simulink model "EVCS_APF_V2G"  (R2024b)
settings: Solver=ode23tb  StartTime=0.0  StopTime=Tstop  MaxStep=1e-5  RelTol=1e-4
PreLoadFcn:
  | model_params
values from neighbouring files (symbols this model uses):
  alpha_lpf = Ts/(tau_lpf+Ts)    (= 0.000125647916761)    [model_params.m]
  Cdc = 3000e-6    (= 0.003)    [model_params.m]
  Cpv = 500e-6    (= 0.0005)    [model_params.m]
  Crf = 20e-6    (= 2e-05)    [model_params.m]
  duty_fix = 0.58    [model_params.m]
  ev_enable = 1    [model_params.m]
  ev_openloop = 0    [model_params.m]
  fgrid = 50    [model_params.m]
  fsw = 10e3    (= 10000)    [model_params.m]
  HB = 0.35    [model_params.m]
  HystSign = -1    [model_params.m]
  Iev_ref = 20    [model_params.m]
  iev_sign = 1    [model_params.m]
  Irr0 = 1000    [model_params.m]
  Irr1 = 700    [model_params.m]
  Ki_dc = 24.6    [model_params.m]
  Ki_ev = 20    [model_params.m]
  Kp_dc = 1.85    [model_params.m]
  Kp_ev = 0.01    [model_params.m]
  Kpu = 1/(VLL*sqrt(2/3))    [model_params.m]
  Lboost = 1.5e-3    (= 0.0015)    [model_params.m]
  Ldc_nl = 20e-3    (= 0.02)    [model_params.m]
  Lev = 5e-3    (= 0.005)    [model_params.m]
  Lf = 1.5e-3    (= 0.0015)    [model_params.m]
  Ls_src = 0.15e-3    (= 0.00015)    [model_params.m]
  Rdc_nl = 10    [model_params.m]
  Rev = 0.2    [model_params.m]
  Rrf = 5    [model_params.m]
  Rs_src = 0.1    [model_params.m]
  t_irr = 0.20    (= 0.2)    [model_params.m]
  t_v2g = 0.30    (= 0.3)    [model_params.m]
  Tcell = 25    [model_params.m]
  Ts = evalin('base','Ts')    [apf_metrics.m]    (also in complexity_analysis.m; harmonic_diagnose.m; model_params.m = 2e-06)
  Vdc_ref = 750    [model_params.m]    (also in pso_tune.m = evalin('base','Vdc_ref'); pso_tune_short.m = evalin('base','Vdc_ref'))
  VLL = 415    [model_params.m]
undefined symbols (not defined in the file or in its folder): Ion, Lithium
libraries: spsSeriesRLCBranchLib x5, spsIGBTDiodeLib x3, spsUniversalBridgeLib x2, spsCurrentMeasurementLib x2, spsThreePhaseSeriesRLCBranchLib x2, spsThreePhaseVIMeasurementLib x2, slpidlib x2, spsVoltageMeasurementLib x2, spsDiodeLib x1, spsBatteryLib x1, spsThreePhaseSourceLib x1, spsThreePhaseSeriesRLCLoadLib x1
settings Model: Creator=dines  LastModifiedBy=dines

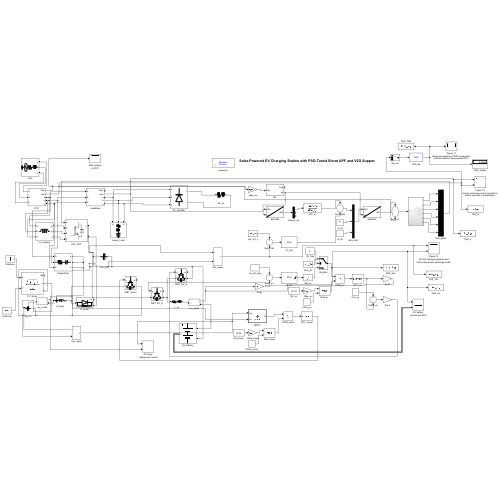
[thumbnail: Simulink's stored preview of the top-level diagram]
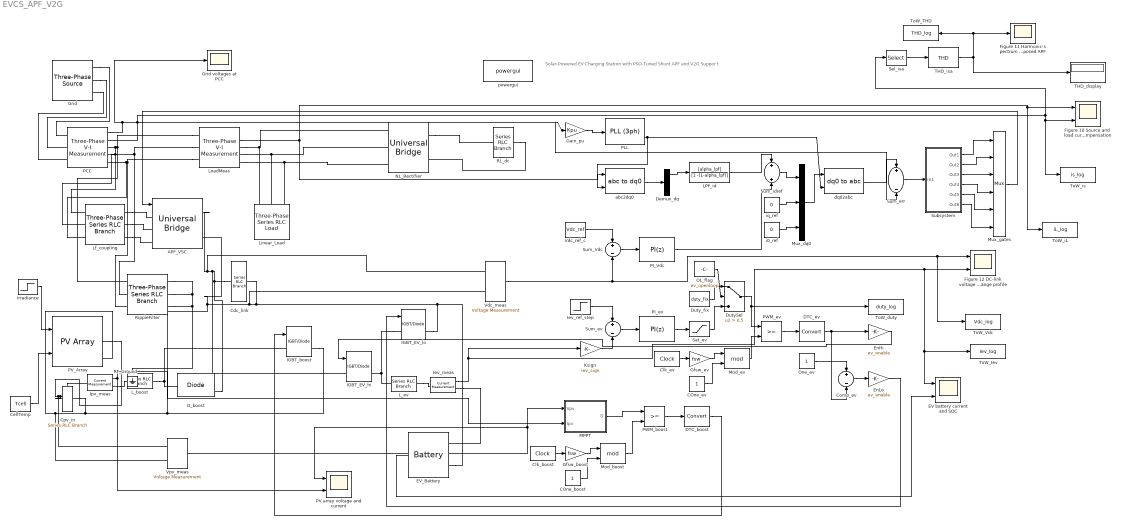
== system EVCS_APF_V2G ==
  note: Solar-Powered EV Charging Station with PSO-Tuned Shunt APF and V2G Suppor t
  APF_VSC : spsUniversalBridgeLib/Universal Bridge  Arms=3  SnubberResistance=1e5  SnubberCapacitance=inf  Device=IGBT / Diodes  Ron=1e-3  Lon=0  ForwardVoltages="[  0  0  ]"  ForwardVoltage=0  GTOparameters=[ 10e-6 , 20e-6 ]  IGBTparameters=[ 1e-6 , 2e-6 ]  Measurements=None  Measurements_2=None  converterType=Rectifier
  COne_boost : Constant
  COne_ev : Constant
  Cdc_link : spsSeriesRLCBranchLib/Series RLC Branch  LConnTagsString=__new0  RConnTagsString=__new0  BranchType=C  Resistance=1  Inductance=1e-3  SetiL0=off  InitialCurrent=0  Capacitance=Cdc  Setx0=off  InitialVoltage=0  Measurements=None
  CellTemp : Constant  Value=Tcell
  Clk_boost : DigitalClock  SampleTime=Ts
  Clk_ev : DigitalClock  SampleTime=Ts
  Comp_ev : Sum  Inputs=+-
  Cpv_in : spsSeriesRLCBranchLib/Series RLC Branch  LConnTagsString=__new0  RConnTagsString=__new0  BranchType=C  Resistance=1  Inductance=1e-3  SetiL0=off  InitialCurrent=0  Capacitance=Cpv  Setx0=off  InitialVoltage=0  Measurements=None
  DTC_boost : DataTypeConversion  SaturateOnIntegerOverflow=off  RndMeth=Floor
  DTC_ev : DataTypeConversion  SaturateOnIntegerOverflow=off  RndMeth=Floor
  D_boost : spsDiodeLib/Diode  Ron=0.001  Lon=0  Vf=0.8  IC=0  UseSnubber=0  Rs=500  Cs=250e-9  Measurements=on
  Demux_dq : Demux  Outputs=3
  DutySel : Switch  Criteria=u2 > Threshold  Threshold=0.5  SaturateOnIntegerOverflow=off  InputSameDT=off
  Duty_fix : Constant  Value=duty_fix
  EV battery current and SOC : Scope  NumInputPorts=2
  EV_Battery : spsBatteryLib/Battery  BatType=Lithium-Ion  NomV=Vbatt  NomQ=Qbatt  SOC=SOC0  Batt_Tr=30  PresetModel=on  MaxQ=40  MinV=270  FullV=419.0354  Dis_rate=17.3913  R=0.09  Normal_OP=36.1739  expZone="[388.9389      1.965217]"
  EnHi : Gain  Gain=ev_enable
  EnLo : Gain  Gain=ev_enable
  Figure 10 Source and load current waveforms before and after compensation : Scope  NumInputPorts=2
  Figure 11 Harmonic-spectrum (THD) comparison with and without the proposed APF : Scope
  Figure 12 DC-link voltage regulation and V2G active-power exchange profile : Scope  NumInputPorts=2
  Gain_pu : Gain  Gain=Kpu
  Gfsw_boost : Gain  Gain=fsw
  Gfsw_ev : Gain  Gain=fsw
  Grid : spsThreePhaseSourceLib/Three-Phase Source  InternalConnection=Yg  VoltagePhases=off  Voltage=VLL  PhaseAngle=0  Voltage_phases=[25e3 25e3 25e3]/sqrt(3)  PhaseAngles_phases=[0 -120 +120]  Frequency=fgrid  NonIdealSource=on  SpecifyImpedance=off  Resistance=Rs_src  Inductance=Ls_src  ShortCircuitLevel=100e6  BaseVoltage=25e3  XRratio=7  BusType=swing  Pref=10e3  Qref=0  Prefabc=[10e3, 10e3, 10e3]  Qrefabc=[0, 0, 0]  Qmin=-inf  Qmax=inf
  Grid voltages at PCC : Scope
  IGBT_EV_hi : spsIGBTDiodeLib/IGBT//Diode  Ron=1e-3  Rs=1e5  Cs=inf  Measurements=on
  IGBT_EV_lo : spsIGBTDiodeLib/IGBT//Diode  Ron=1e-3  Rs=1e5  Cs=inf  Measurements=on
  IGBT_boost : spsIGBTDiodeLib/IGBT//Diode  Ron=1e-3  Rs=1e5  Cs=inf  Measurements=on
  Iev_meas : spsCurrentMeasurementLib/Current Measurement  PhasorSimulation=off  OutputType=Complex  PSBequivalent=0
  Iev_ref_step : Step  Time=t_v2g  Before=Iev_ref  After=-Iev_ref  SampleTime=0
  Ipv_meas : spsCurrentMeasurementLib/Current Measurement  PhasorSimulation=off  OutputType=Complex  PSBequivalent=0
  Irradiance : Step  Time=t_irr  Before=Irr0  After=Irr1  SampleTime=0
  Ksign : Gain  Gain=iev_sign
  LPF_id : DiscreteTransferFcn  Numerator=[alpha_lpf]  Denominator=[1 -(1-alpha_lpf)]  SampleTime=Ts
  L_boost : spsSeriesRLCBranchLib/Series RLC Branch  LConnTagsString=__new0  RConnTagsString=__new0  BranchType=L  Resistance=1  Inductance=Lboost  SetiL0=off  InitialCurrent=0  Capacitance=1e-6  Setx0=off  InitialVoltage=0  Measurements=None
  L_ev : spsSeriesRLCBranchLib/Series RLC Branch  LConnTagsString=__new0  RConnTagsString=__new0  BranchType=RL  Resistance=Rev  Inductance=Lev  SetiL0=off  InitialCurrent=0  Capacitance=1e-6  Setx0=off  InitialVoltage=0  Measurements=None
  Lf_coupling : spsThreePhaseSeriesRLCBranchLib/Three-Phase Series RLC Branch  LConnTagsString=A|B|C  RConnTagsString=A|B|C  BranchType=L  Resistance=1  Inductance=Lf  Capacitance=1e-6  Measurements=None
  Linear_Load : spsThreePhaseSeriesRLCLoadLib/Three-Phase Series RLC Load  LConnTagsString=A|B|C  Configuration=Y (grounded)  NominalVoltage=VLL  Vabc=[1e3 1e3 1e3]  Vabcp=[1e3 1e3 1e3]  NominalFrequency=fgrid  UnbalancedPower=off  ActivePower=Plin  InductivePower=100  CapacitivePower=100  Pabc=[10e3 9e3 11e3]  QLabc=[100 90 110]  QCabc=[100 90 110]  Pabcp=[10e3 9e3 11e3]  QLabcp=[100 90 110]  QCabcp=[100 90 110]  Measurements=None  LoadType=constant Z
  LoadMeas : spsThreePhaseVIMeasurementLib/Three-Phase V-I Measurement  VoltageMeasurement=phase-to-ground  SetLabelV=off  LabelV=Vabc  Vpu=off  VpuLL=off  CurrentMeasurement=yes  SetLabelI=off  LabelI=Iabc  Ipu=off  Pbase=100e6  Vbase=500e3  OutputType=Complex  PhasorSimulation=off  PSBequivalent=0
  MPPT : MATLAB Function  TreatAsAtomicUnit=on
  Mod_boost : Math  Operator=mod
  Mod_ev : Math  Operator=mod
  Mux_dq0 : Mux  Inputs=3
  Mux_gates : Mux  Inputs=6
  NL_Rectifier : spsUniversalBridgeLib/Universal Bridge  Arms=3  SnubberResistance=1e5  SnubberCapacitance=inf  Device=Diodes  Ron=1e-3  Lon=0  ForwardVoltages="[  0  0  ]"  ForwardVoltage=0  GTOparameters=[ 10e-6 , 20e-6 ]  IGBTparameters=[ 1e-6 , 2e-6 ]  Measurements=None  Measurements_2=None  converterType=Rectifier
  OL_flag : Constant  Value=ev_openloop
  One_ev : Constant
  PCC : spsThreePhaseVIMeasurementLib/Three-Phase V-I Measurement  VoltageMeasurement=phase-to-ground  SetLabelV=off  LabelV=Vabc  Vpu=off  VpuLL=off  CurrentMeasurement=yes  SetLabelI=off  LabelI=Iabc  Ipu=off  Pbase=100e6  Vbase=500e3  OutputType=Complex  PhasorSimulation=off  PSBequivalent=0
  PI_Vdc : slpidlib/PID Controller  Controller=PI  Form=Parallel  TimeDomain=Discrete-time  UseExternalTs=off  SampleTime=Ts  IntegratorMethod=Forward Euler  FilterMethod=Forward Euler  ControllerParametersSource=internal  P=Kp_dc  I=Ki_dc  UseKiTs=off  D=0  UseExternalDerivativeSource=off  N=100  UseFilter=on  TunerSelectOption=Transfer Function Based (PID Tuner App)  InitialConditionSource=internal  InitialConditionForIntegrator=0  InitialConditionForFilter=0  DifferentiatorICPrevScaledInput=0  ExternalReset=none  TrackingMode=off  Kt=1  LimitOutput=off  SatLimitsSource=internal  UpperSaturationLimit=inf  LowerSaturationLimit=-inf  LinearizeAsGain=on  AntiWindupMode=none  Kb=1  LimitIntegrator=off  UpperIntegratorSaturationLimit=inf  LowerIntegratorSaturationLimit=-inf  POutMin=[]  POutMax=[]  IOutMin=[]  IOutMax=[]  DOutMin=[]  DOutMax=[]  NOutMin=[]  NOutMax=[]  SumOutMin=[]  SumOutMax=[]  SaturationOutMin=[]  SaturationOutMax=[]  PParamMin=[]  PParamMax=[]  IParamMin=[]  IParamMax=[]  DParamMin=[]  DParamMax=[]  NParamMin=[]  NParamMax=[]  KbParamMin=[]  KbParamMax=[]  KtParamMin=[]  KtParamMax=[]  KbOutMin=[]  KbOutMax=[]  KtOutMin=[]  KtOutMax=[]  IntegratorOutMin=[]  IntegratorOutMax=[]  FilterOutMin=[]  FilterOutMax=[]  SumI1OutMin=[]  SumI1OutMax=[]  SumI2OutMin=[]  SumI2OutMax=[]  SumI3OutMin=[]  SumI3OutMax=[]  SumI4OutMin=[]  SumI4OutMax=[]  SumDOutMin=[]  SumDOutMax=[]  DifferentiatorOutMin=[]  DifferentiatorOutMax=[]  FilterDiffOutCoefMin=[]  FilterDiffOutCoefMax=[]  ReciprocalOutMin=[]  ReciprocalOutMax=[]  SumDenOutMin=[]  SumDenOutMax=[]  SumNumOutMin=[]  SumNumOutMax=[]  DivideOutMin=[]  DivideOutMax=[]  UdiffTsProdOutMin=[]  UdiffTsProdOutMax=[]  NTsProdOutMin=[]  NTsProdOutMax=[]  UintegralTsProdOutMin=[]  UintegralTsProdOutMax=[]  UngainTsProdOutMin=[]  UngainTsProdOutMax=[]  ClampingZeroOutDataTypeStr=Inherit: Inherit via back propagation  ClampingZeroOutMin=[]  ClampingZeroOutMax=[]  FilterDenConstantOutDataTypeStr=Inherit: Inherit via back propagation  FilterDenConstantOutMin=[]  FilterDenConstantOutMax=[]  PCopyOutDataTypeStr=Inherit: Inherit via back propagation  PCopyOutMin=[]  PCopyOutMax=[]  NCopyOutDataTypeStr=Inherit: Inherit via back propagation  NCopyOutMin=[]  NCopyOutMax=[]  IntegratorContinuousStateAttributes=''  IntegratorStateMustResolveToSignalObject=off  IntegratorRTWStateStorageClass=Auto  FilterContinuousStateAttributes=''  FilterStateMustResolveToSignalObject=off  FilterRTWStateStorageClass=Auto  ParallelPVariant=InternalParameters  IdealPVariant=Disabled  IVariant=InternalParameters  DVariant=Disabled  IntegratorVariant=Discrete  SatVariant=Disabled  AWVariant=Passthrough  PCopyVariant=Disabled  TRVariant=Disabled  FdbkBlocksVariant=Forward  IdealPFdbkVariant=Disabled  SatFdbkVariant=Disabled  DerivativeFilterVariant=Disabled  NVariant=Disabled  NCopyVariant=Disabled_SignalSpec  FilterICVariant=Disabled  IntegratorICVariant=InternalICs  ExternalResetVariant=Disabled  TRSumVariant=Passthrough  SumFdbkVariant=Disabled  SumVariant=Sum_PI  TsampFilterVariant=InternalTs  TsampNgainVariant=Passthrough  TsampIntegralVariant=Disabled_SignalSpec  ExternalSaturationOutDataTypeStr=Inherit: Same as second input  DerivativeSourceVariant=Disabled  PreIntVariant=InternalPreInt
  PI_ev : slpidlib/PID Controller  Controller=PI  Form=Parallel  TimeDomain=Discrete-time  UseExternalTs=off  SampleTime=Ts  IntegratorMethod=Forward Euler  FilterMethod=Forward Euler  ControllerParametersSource=internal  P=Kp_ev  I=Ki_ev  UseKiTs=off  D=0  UseExternalDerivativeSource=off  N=100  UseFilter=on  TunerSelectOption=Transfer Function Based (PID Tuner App)  InitialConditionSource=internal  InitialConditionForIntegrator=duty0  InitialConditionForFilter=0  DifferentiatorICPrevScaledInput=0  ExternalReset=none  TrackingMode=off  Kt=1  LimitOutput=on  SatLimitsSource=internal  UpperSaturationLimit=0.95  LowerSaturationLimit=0.05  LinearizeAsGain=on  AntiWindupMode=clamping  Kb=1  LimitIntegrator=off  UpperIntegratorSaturationLimit=inf  LowerIntegratorSaturationLimit=-inf  POutMin=[]  POutMax=[]  IOutMin=[]  IOutMax=[]  DOutMin=[]  DOutMax=[]  NOutMin=[]  NOutMax=[]  SumOutMin=[]  SumOutMax=[]  SaturationOutMin=[]  SaturationOutMax=[]  PParamMin=[]  PParamMax=[]  IParamMin=[]  IParamMax=[]  DParamMin=[]  DParamMax=[]  NParamMin=[]  NParamMax=[]  KbParamMin=[]  KbParamMax=[]  KtParamMin=[]  KtParamMax=[]  KbOutMin=[]  KbOutMax=[]  KtOutMin=[]  KtOutMax=[]  IntegratorOutMin=[]  IntegratorOutMax=[]  FilterOutMin=[]  FilterOutMax=[]  SumI1OutMin=[]  SumI1OutMax=[]  SumI2OutMin=[]  SumI2OutMax=[]  SumI3OutMin=[]  SumI3OutMax=[]  SumI4OutMin=[]  SumI4OutMax=[]  SumDOutMin=[]  SumDOutMax=[]  DifferentiatorOutMin=[]  DifferentiatorOutMax=[]  FilterDiffOutCoefMin=[]  FilterDiffOutCoefMax=[]  ReciprocalOutMin=[]  ReciprocalOutMax=[]  SumDenOutMin=[]  SumDenOutMax=[]  SumNumOutMin=[]  SumNumOutMax=[]  DivideOutMin=[]  DivideOutMax=[]  UdiffTsProdOutMin=[]  UdiffTsProdOutMax=[]  NTsProdOutMin=[]  NTsProdOutMax=[]  UintegralTsProdOutMin=[]  UintegralTsProdOutMax=[]  UngainTsProdOutMin=[]  UngainTsProdOutMax=[]  ClampingZeroOutDataTypeStr=Inherit: Inherit via back propagation  ClampingZeroOutMin=[]  ClampingZeroOutMax=[]  FilterDenConstantOutDataTypeStr=Inherit: Inherit via back propagation  FilterDenConstantOutMin=[]  FilterDenConstantOutMax=[]  PCopyOutDataTypeStr=Inherit: Inherit via back propagation  PCopyOutMin=[]  PCopyOutMax=[]  NCopyOutDataTypeStr=Inherit: Inherit via back propagation  NCopyOutMin=[]  NCopyOutMax=[]  IntegratorContinuousStateAttributes=''  IntegratorStateMustResolveToSignalObject=off  IntegratorRTWStateStorageClass=Auto  FilterContinuousStateAttributes=''  FilterStateMustResolveToSignalObject=off  FilterRTWStateStorageClass=Auto  ParallelPVariant=InternalParameters  IdealPVariant=Disabled  IVariant=InternalParameters  DVariant=Disabled  IntegratorVariant=Discrete  SatVariant=Enabled  AWVariant=DiscClampingParallel  PCopyVariant=Disabled  TRVariant=Disabled  FdbkBlocksVariant=Forward  IdealPFdbkVariant=Disabled  SatFdbkVariant=Disabled  DerivativeFilterVariant=Disabled  NVariant=Disabled  NCopyVariant=Disabled_SignalSpec  FilterICVariant=Disabled  IntegratorICVariant=InternalICs  ExternalResetVariant=Disabled  TRSumVariant=Passthrough  SumFdbkVariant=Disabled  SumVariant=Sum_PI  TsampFilterVariant=InternalTs  TsampNgainVariant=Passthrough  TsampIntegralVariant=Disabled_SignalSpec  ExternalSaturationOutDataTypeStr=Inherit: Same as second input  DerivativeSourceVariant=Disabled  PreIntVariant=InternalPreInt
  PLL : spsPLL3phLib/PLL (3ph)  Fmin=45  Par_Init=[0, 60]  ParK=[180, 3200, 1]  TcD=1e-4  MaxRateChangeFreq=12  FilterCutOffFreq=25  Ts=Ts  AGC=on
  PV array voltage and current : Scope  NumInputPorts=2
  PV_Array : spsPVArrayLib/PV Array  Npar=Npar  Nser=Nser  PlotType=array @ 1000 W/m2 & specified temperatures  S_vec="[ 1000  500  100 ]"  Temp_C_vec="[ 45 25  ]"  ModuleName=SunPower SPR-305E-WHT-D  PlotWhenSelected=off  Pm=305.226  Ncell=96  Voc=64.2  Isc=5.96  Vm=54.7  Im=5.58  beta_Voc_pc=-0.2727  alpha_Isc_pc=0.061745  beta_Voc=-0.17507  alpha_Isc=0.00368  IL=5.9657  I0=6.3076e-12  nI=0.94489  Rsh=393.2054  Rs=0.37428  RobustModel=off  RobustCellTemperature=313.3991  BAL=on  Tc=1e-6  Tfilter=5e-5
  PWM_boost : RelationalOperator  OutDataTypeStr=boolean  RndMeth=Simplest  InputSameDT=off
  PWM_ev : RelationalOperator  OutDataTypeStr=boolean  RndMeth=Simplest  InputSameDT=off
  RF_Ground : spsGroundLib/Ground  LConnTagsString=a
  RL_dc : spsSeriesRLCBranchLib/Series RLC Branch  LConnTagsString=__new0  RConnTagsString=__new0  BranchType=RL  Resistance=Rdc_nl  Inductance=Ldc_nl  SetiL0=off  InitialCurrent=0  Capacitance=1e-6  Setx0=off  InitialVoltage=0  Measurements=None
  RippleFilter : spsThreePhaseSeriesRLCBranchLib/Three-Phase Series RLC Branch  LConnTagsString=A|B|C  RConnTagsString=A|B|C  BranchType=RC  Resistance=Rrf  Inductance=1e-3  Capacitance=Crf  Measurements=None
  Sat_ev : Saturate  UpperLimit=0.95  LowerLimit=0.05
  Sel_isa : Selector  InputPortWidth=3  IndexOptions=Index vector (dialog)  Indices=1  OutputSizes=1
  Subsystem : Subsystem
  Sum_Vdc : Sum  Inputs=+-
  Sum_err : Sum  Inputs=+-
  Sum_ev : Sum  Inputs=+-
  Sum_idref : Sum
  THD_display : Display
  THD_isa : spsTHDLib/THD  Freq=fgrid  Ts=0
  ToW_Iev : ToWorkspace  VariableName=Iev_log  SaveFormat=Timeseries  SampleTime=-1
  ToW_THD : ToWorkspace  VariableName=THD_log  SaveFormat=Timeseries  SampleTime=-1
  ToW_Vdc : ToWorkspace  VariableName=Vdc_log  SaveFormat=Timeseries  SampleTime=-1
  ToW_duty : ToWorkspace  VariableName=duty_log  SaveFormat=Timeseries  SampleTime=-1
  ToW_iL : ToWorkspace  VariableName=iL_log  SaveFormat=Timeseries  SampleTime=-1
  ToW_is : ToWorkspace  VariableName=is_log  SaveFormat=Timeseries  SampleTime=-1
  Vdc_meas : spsVoltageMeasurementLib/Voltage Measurement  PhasorSimulation=off  OutputType=Complex  PSBequivalent=0
  Vdc_ref_c : Constant  Value=Vdc_ref
  Vpv_meas : spsVoltageMeasurementLib/Voltage Measurement  PhasorSimulation=off  OutputType=Complex  PSBequivalent=0
  abc2dq0 : spsabctodq0Lib/abc to dq0  Alignment=90 degrees behind phase A axis
  dq02abc : spsdq0toabcLib/dq0 to abc  Alignment=90 degrees behind phase A axis
  i0_ref : Constant  Value=0
  iq_ref : Constant  Value=0
  powergui : sps_lib/powergui  Priority=1  SimulationMode=Discrete  SampleTime=Ts  frequency=60  Iterations=50  frequencyindice=0  Pbase=100e6  ErrMax=1e-4  UnitsV=kV  UnitsW=MW  buscounter=0  FunctionMessages=off  echomessages=off  EnableUseOfTLC=off  CurrentSourceSwitches=off  DisableSnubberDevices=off  DisableRonSwitches=off  DisableVfSwitches=off  DisplayEquations=off  AutomaticDiscreteSolvers=off  SolverType=Tustin/Backward Euler (TBE)  Interpol=off  ExternalGateDelay=off  methode=off  Ts=100  x0status=blocks  SPID=on  SwTol=0  HookPort=off  NonlinearTolerance=1e-4  nMaxIteration=100  ContinueOnMaxIteration=off  RestoreLinks=warning  ResistiveCurrentMeasurement=off  Frange=[0:2:500]  Ylog=off  Xlog=on  ShowGrid=off  save=off  variable=ZData  structure=0  ZoomFFT=off  StartTime=0.0  cycles=1  DisplayStyle=1  fundamental=60  FreqAxis=off  MaxFrequency=1000  frequencyindicesteady=1  RmsSteady=1  display=off
  wires:
  Irradiance/1 -> PV_Array/1
  CellTemp/1 -> PV_Array/2
  PCC/1 -> Gain_pu/1, Grid voltages at PCC/1
  Gain_pu/1 -> PLL/1
  PLL/2 -> abc2dq0/2, dq02abc/2
  LoadMeas/2 -> Figure 10 Source and load current waveforms before and after compensation/1, ToW_iL/1, abc2dq0/1
  abc2dq0/1 -> Demux_dq/1
  Demux_dq/1 -> LPF_id/1
  Vdc_ref_c/1 -> Sum_Vdc/1
  Vdc_meas/1 -> Figure 12 DC-link voltage regulation and V2G active-power exchange profile/1, ToW_Vdc/1, Sum_Vdc/2
  Sum_Vdc/1 -> PI_Vdc/1
  LPF_id/1 -> Sum_idref/1
  PI_Vdc/1 -> Sum_idref/2
  Sum_idref/1 -> Mux_dq0/1
  iq_ref/1 -> Mux_dq0/2
  i0_ref/1 -> Mux_dq0/3
  Mux_dq0/1 -> dq02abc/1
  dq02abc/1 -> Sum_err/1
  PCC/2 -> Sel_isa/1, ToW_is/1, Figure 10 Source and load current waveforms before and after compensation/2, Sum_err/2
  Mux_gates/1 -> APF_VSC/1
  Vpv_meas/1 -> MPPT/1(Vpv), PV array voltage and current/1
  Ipv_meas/1 -> MPPT/2(Ipv), PV array voltage and current/2
  MPPT/1(D) -> PWM_boost/1
  Clk_boost/1 -> Gfsw_boost/1
  Gfsw_boost/1 -> Mod_boost/1
  COne_boost/1 -> Mod_boost/2
  Mod_boost/1 -> PWM_boost/2
  PWM_boost/1 -> DTC_boost/1
  DTC_boost/1 -> IGBT_boost/1
  Iev_ref_step/1 -> Sum_ev/1
  Iev_meas/1 -> ToW_Iev/1, EV battery current and SOC/1, Figure 12 DC-link voltage regulation and V2G active-power exchange profile/2, Ksign/1
  Ksign/1 -> Sum_ev/2
  Sum_ev/1 -> PI_ev/1
  PI_ev/1 -> Sat_ev/1
  Duty_fix/1 -> DutySel/1
  OL_flag/1 -> DutySel/2
  Sat_ev/1 -> DutySel/3
  DutySel/1 -> PWM_ev/1, ToW_duty/1
  Clk_ev/1 -> Gfsw_ev/1
  Gfsw_ev/1 -> Mod_ev/1
  COne_ev/1 -> Mod_ev/2
  Mod_ev/1 -> PWM_ev/2
  PWM_ev/1 -> DTC_ev/1
  One_ev/1 -> Comp_ev/1
  DTC_ev/1 -> EnHi/1, Comp_ev/2
  Comp_ev/1 -> EnLo/1
  EnHi/1 -> IGBT_EV_hi/1
  EnLo/1 -> IGBT_EV_lo/1
  Sel_isa/1 -> THD_isa/1
  THD_isa/1 -> ToW_THD/1, Figure 11 Harmonic-spectrum (THD) comparison with and without the proposed APF/1, THD_display/1
  EV_Battery/1 -> EV battery current and SOC/2
  Sum_err/1 -> Subsystem/1(In1)
  Subsystem/1(Out1) -> Mux_gates/1
  Subsystem/2(Out2) -> Mux_gates/2
  Subsystem/3(Out3) -> Mux_gates/3
  Subsystem/4(Out4) -> Mux_gates/4
  Subsystem/5(Out5) -> Mux_gates/5
  Subsystem/6(Out6) -> Mux_gates/6
  connections:
  Grid/RConn1 -- PCC/LConn1
  Grid/RConn2 -- PCC/LConn2
  Grid/RConn3 -- PCC/LConn3
  LoadMeas/LConn1 -- PCC/RConn1 -- Lf_coupling/LConn1 -- RippleFilter/LConn1
  LoadMeas/LConn2 -- PCC/RConn2 -- Lf_coupling/LConn2 -- RippleFilter/LConn2
  LoadMeas/LConn3 -- PCC/RConn3 -- Lf_coupling/LConn3 -- RippleFilter/LConn3
  LoadMeas/RConn1 -- NL_Rectifier/LConn1 -- Linear_Load/LConn1
  LoadMeas/RConn2 -- NL_Rectifier/LConn2 -- Linear_Load/LConn2
  LoadMeas/RConn3 -- NL_Rectifier/LConn3 -- Linear_Load/LConn3
  NL_Rectifier/RConn1 -- RL_dc/LConn1
  RL_dc/RConn1 -- NL_Rectifier/RConn2
  Lf_coupling/RConn1 -- APF_VSC/LConn1
  Lf_coupling/RConn2 -- APF_VSC/LConn2
  Lf_coupling/RConn3 -- APF_VSC/LConn3
  Cdc_link/LConn1 -- APF_VSC/RConn1 -- Vdc_meas/LConn1 -- IGBT_EV_hi/LConn1 -- D_boost/RConn1
  Cdc_link/RConn1 -- EV_Battery/LConn2 -- IGBT_EV_lo/RConn1 -- APF_VSC/RConn2 -- PV_Array/RConn2 -- Vpv_meas/LConn2 -- Cpv_in/RConn1 -- IGBT_boost/RConn1 -- Vdc_meas/LConn2
  Cpv_in/LConn1 -- PV_Array/RConn1 -- Vpv_meas/LConn1 -- Ipv_meas/LConn1
  Ipv_meas/RConn1 -- L_boost/LConn1
  D_boost/LConn1 -- IGBT_boost/LConn1 -- L_boost/RConn1
  IGBT_EV_lo/LConn1 -- L_ev/LConn1 -- IGBT_EV_hi/RConn1
  L_ev/RConn1 -- Iev_meas/LConn1
  Iev_meas/RConn1 -- EV_Battery/LConn1
  RippleFilter/RConn1 -- RF_Ground/LConn1 -- RippleFilter/RConn3 -- RippleFilter/RConn2

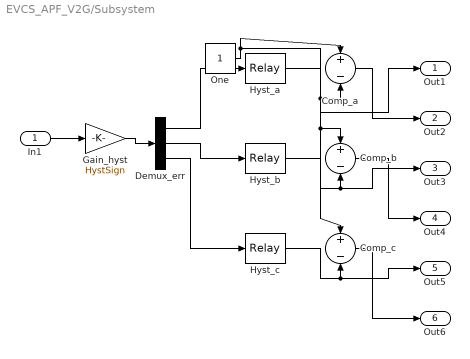
== system EVCS_APF_V2G/Subsystem ==
  In1 : Inport
  Comp_a : Sum  Inputs=+-
  Comp_b : Sum  Inputs=+-
  Comp_c : Sum  Inputs=+-
  Demux_err : Demux  Outputs=3
  Gain_hyst : Gain  Gain=HystSign
  Hyst_a : Relay  OnSwitchValue=HB/2  OffSwitchValue=-HB/2
  Hyst_b : Relay  OnSwitchValue=HB/2  OffSwitchValue=-HB/2
  Hyst_c : Relay  OnSwitchValue=HB/2  OffSwitchValue=-HB/2
  One : Constant
  Out1 : Outport
  Out2 : Outport  Port=2
  Out3 : Outport  Port=3
  Out4 : Outport  Port=4
  Out5 : Outport  Port=5
  Out6 : Outport  Port=6
  wires:
  Hyst_a/1 -> Out1/1, Comp_a/2
  Demux_err/3 -> Hyst_c/1
  One/1 -> Comp_b/1, Comp_c/1, Comp_a/1
  Demux_err/1 -> Hyst_a/1
  Demux_err/2 -> Hyst_b/1
  Gain_hyst/1 -> Demux_err/1
  Hyst_c/1 -> Out5/1, Comp_c/2
  Hyst_b/1 -> Out3/1, Comp_b/2
  In1/1 -> Gain_hyst/1
  Comp_c/1 -> Out6/1
  Comp_a/1 -> Out2/1
  Comp_b/1 -> Out4/1

== matlab function EVCS_APF_V2G/MPPT ==
  data: Vpv input; D output; Ipv input
function D = pando(Vpv, Ipv)
%#codegen
% Perturb & Observe MPPT (Eq. 3). Updates every 400 samples (~2 ms @ Ts=5e-6).
persistent Dold Pold Vold cnt
if isempty(Dold), Dold = 0.4; Pold = 0; Vold = 0; cnt = 0; end
cnt = cnt + 1;
D = Dold;
if cnt >= 400
    cnt = 0;
    P  = Vpv*Ipv;
    dP = P - Pold;   dV = Vpv - Vold;   dD = 2e-3;
    if abs(dP) > 1e-3
        if dP > 0
            if dV > 0, D = Dold - dD; else, D = Dold + dD; end
        else
            if dV > 0, D = Dold + dD; else, D = Dold - dD; end
        end
    end
    D = min(max(D, 0.05), 0.85);
    Pold = P;  Vold = Vpv;  Dold = D;
end
